simulink model "Lab6"  (R2012b)
settings: Solver=ode1  StartTime=0.0  StopTime=inf  FixedStep=0.002  RelTol=1e-3
undefined symbols (not defined in the file): HIL
libraries: quarc_library x5
settings Model: ExtModeTrigDuration=5000  Creator=paichihyun  LastModifiedBy=paichihyun
settings SolverCC: PositivePriorityOrder=on
settings RTWCC: SystemTargetFile=quarc_win64.tlc  TemplateMakefile=quarc_default_tmf  Description=QUARC Win64 Target  ProcessScript=quarc_win64_make_rtw_hook
settings STFCustomTargetCC: TargetPreCompLibLocation=C:\PROGRA~3\QUARC\lib\2012b\win64\release  CodeReplacementLibrary=ANSI_C  GeneratePreprocessorConditionals=Disable all  CombineOutputUpdateFcns=on  GRTInterface=off  SystemTargetFile=quarc_win64.tlc
settings GRTTargetCC: TargetPreCompLibLocation=C:\PROGRA~3\QUARC\lib\2012b\win64\release  ParMdlRefBuildCompliant=off  CompOptLevelCompliant=off  ConcurrentExecutionCompliant=off  MatFileLogging=off  ExtMode=on  ExtModeMexFile=quarc_comm

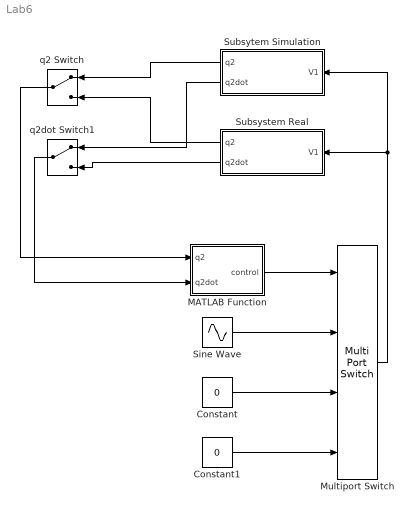
== system Lab6 ==
  Constant : Constant  Value=0
  Constant1 : Constant  Value=0
  MATLAB Function : MATLAB Function  TreatAsAtomicUnit=on
  Multiport Switch : MultiPortSwitch
  Sine Wave : Sin  SampleTime=0
  Subsystem Real : Subsystem
  Subsytem Simulation : Subsystem
  q2 Switch : ManualSwitch
  q2dot Switch1 : ManualSwitch
  wires:
  MATLAB Function/1(control) -> Multiport Switch/1
  Constant/1 -> Multiport Switch/3
  Sine Wave/1 -> Multiport Switch/2
  Constant1/1 -> Multiport Switch/4
  Multiport Switch/1 -> Subsystem Real/1(V1), Subsytem Simulation/1(V1)
  Subsytem Simulation/1(q2) -> q2 Switch/1
  Subsystem Real/1(q2) -> q2 Switch/2
  Subsytem Simulation/2(q2dot) -> q2dot Switch1/1
  Subsystem Real/2(q2dot) -> q2dot Switch1/2
  q2 Switch/1 -> MATLAB Function/1(q2)
  q2dot Switch1/1 -> MATLAB Function/2(q2dot)

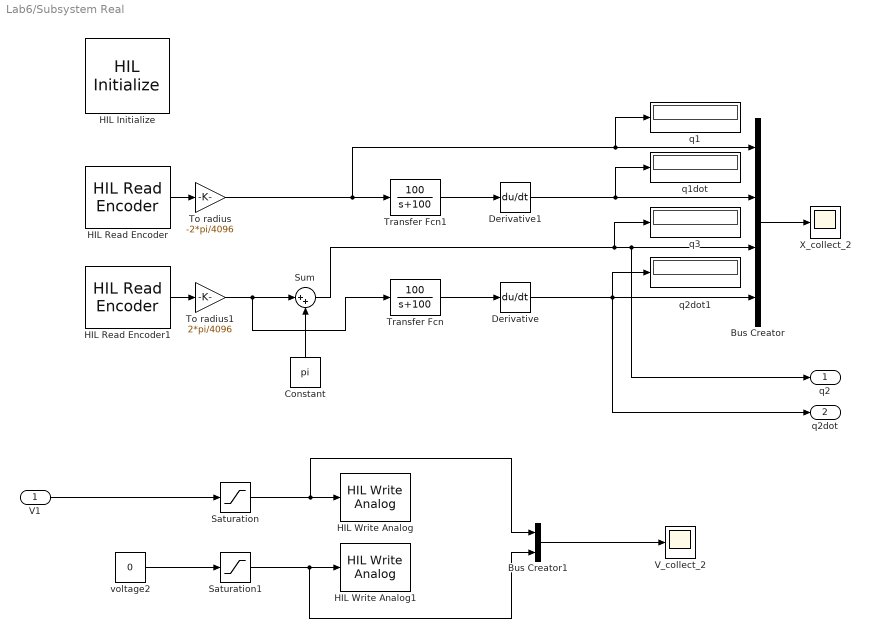
== system Lab6/Subsystem Real ==
  V1 : Inport
  Bus Creator : BusCreator
  Bus Creator1 : BusCreator  Inputs=2
  Constant : Constant  Value=pi
  Derivative : Derivative
  Derivative1 : Derivative
  HIL Initialize : quarc_library/Data Acquisition/Generic/Configuration/HIL Initialize  Priority=-99  object_name=HIL-1  board_type=q2_usb  board_number=0  board_options=d0=digital;d1=digital;led=auto;update_rate=normal;decimation=1  exclusive=off  active=off  hardware_clocks=[0]  clock_modes=[]  initial_clock_frequencies=[]  set_clock_params_at_start=off  set_clock_params_at_switch_in=off  set_clock_frequencies_at_start=off  set_clock_frequencies_at_switch_in=off  analog_input_channels=[0:1]  analog_input_maximums=10  analog_input_minimums=-10  set_analog_input_params_at_start=on  set_analog_input_params_at_switch_in=off  analog_output_channels=[0:1]  analog_output_maximums=10  analog_output_minimums=-10  initial_analog_outputs=[0]  final_analog_outputs=[0]  watchdog_analog_outputs=0  set_analog_output_params_at_start=on  set_analog_output_params_at_switch_in=off  set_analog_outputs_at_start=on  set_analog_outputs_at_switch_in=off  set_analog_outputs_at_terminate=on  set_analog_outputs_at_switch_out=off  set_analog_outputs_on_watchdog=off  digital_input_channels=[]  digital_output_channels=[]  digital_output_configuration=[]  initial_digital_outputs=[1]  final_digital_outputs=[1]  watchdog_digital_outputs=[1]  set_digital_output_params_at_start=off  set_digital_output_params_at_switch_in=off  set_digital_outputs_at_start=on  set_digital_outputs_at_switch_in=off  set_digital_outputs_at_terminate=on  set_digital_outputs_at_switch_out=off  set_digital_outputs_on_watchdog=off  encoder_channels=[0:1]  quadrature=[4]  encoder_filter_frequency=[]  initial_encoder_counts=[0]  set_encoder_params_at_start=on  set_encoder_params_at_switch_in=off  set_encoder_counts_at_start=on  set_encoder_counts_at_switch_in=off  pwm_channels=[]  pwm_modes=[0]  pwm_frequency=1/0.020  pwm_configuration=[]  pwm_alignment=[]  pwm_polarity=[]  pwm_leading_deadband=[]  pwm_trailing_deadband=[]  initial_pwm_outputs=[0]  final_pwm_outputs=[0]  watchdog_pwm_outputs=[0]  set_pwm_params_at_start=on  set_pwm_params_at_switch_in=off  set_pwm_outputs_at_start=on  set_pwm_outputs_at_switch_in=off  set_pwm_outputs_at_terminate=on  set_pwm_outputs_at_switch_out=off  set_pwm_outputs_on_watchdog=off  other_output_channels=[]  initial_other_outputs=[]  final_other_outputs=[]  watchdog_other_outputs=[]  set_other_outputs_at_start=off  set_other_outputs_at_switch_in=off  set_other_outputs_at_terminate=off  set_other_outputs_at_switch_out=off  set_other_outputs_on_watchdog=off
  HIL Read Encoder : quarc_library/Data Acquisition/Generic/Immediate I//O/HIL Read Encoder  object_name=HIL-1  channels=0  sample_time=qc_get_step_size  active=on  vector_output=off  data_type_mode=Inherit via back propagation  data_type=double
  HIL Read Encoder1 : quarc_library/Data Acquisition/Generic/Immediate I//O/HIL Read Encoder  object_name=HIL-1  channels=1  sample_time=qc_get_step_size  active=on  vector_output=off  data_type_mode=Inherit via back propagation  data_type=double
  HIL Write Analog : quarc_library/Data Acquisition/Generic/Immediate I//O/HIL Write Analog  object_name=HIL-1  channels=0  sample_time=-1  active=off  vector_input=off
  HIL Write Analog1 : quarc_library/Data Acquisition/Generic/Immediate I//O/HIL Write Analog  object_name=HIL-1  channels=1  sample_time=-1  active=off  vector_input=off
  Saturation : Saturate  UpperLimit=10  LowerLimit=-10
  Saturation1 : Saturate  UpperLimit=10  LowerLimit=-10
  Sum : Sum  Inputs=|++
  To radius : Gain  Gain=-2*pi/4096
  To radius1 : Gain  Gain=2*pi/4096
  Transfer Fcn : TransferFcn  Numerator=[100]  Denominator=[1 100]
  Transfer Fcn1 : TransferFcn  Numerator=[100]  Denominator=[1 100]
  V_collect_2 : Scope
      settings: SaveName=V_collect_  SampleInput=on  SampleTime=0.001
  "X_collect_2 " : Scope
      settings: SaveName=X_collect_  SampleInput=on  SampleTime=0.001
  q1 : Display
  q1dot : Display
  q2dot1 : Display
  q3 : Display
  voltage2 : Constant  Value=0
  q2 : Outport
  q2dot : Outport  Port=2
  wires:
  Transfer Fcn/1 -> Derivative/1
  HIL Read Encoder/1 -> To radius/1
  HIL Read Encoder1/1 -> To radius1/1
  Constant/1 -> Sum/2
  To radius1/1 -> Transfer Fcn/1, Sum/1
  Transfer Fcn1/1 -> Derivative1/1
  To radius/1 -> q1/1, Bus Creator/1, Transfer Fcn1/1
  Sum/1 -> q2/1, Bus Creator/3, q3/1
  Derivative/1 -> q2dot/1, Bus Creator/4, q2dot1/1
  Derivative1/1 -> Bus Creator/2, q1dot/1
  Bus Creator/1 -> "X_collect_2 "/1
  Saturation/1 -> Bus Creator1/1, HIL Write Analog/1
  Saturation1/1 -> Bus Creator1/2, HIL Write Analog1/1
  voltage2/1 -> Saturation1/1
  Bus Creator1/1 -> V_collect_2/1
  V1/1 -> Saturation/1

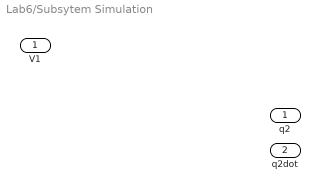
== system Lab6/Subsytem Simulation ==
  V1 : Inport
  q2 : Outport
  q2dot : Outport  Port=2

== matlab function Lab6/MATLAB Function ==
  data: q2 input; control output; q2dot input
function control = fcn(q2, q2dot)
%#codegen

control = 0;
